simulink model "Silva22211767SL"  (R2025b)
settings: Solver=ode15s  StartTime=0.0  StopTime=100  RelTol=1e-3
settings Model: Creator=karla  LastModifiedBy=karla
settings DataIOCC: ReturnWorkspaceOutputs=off  TimeSaveName=t

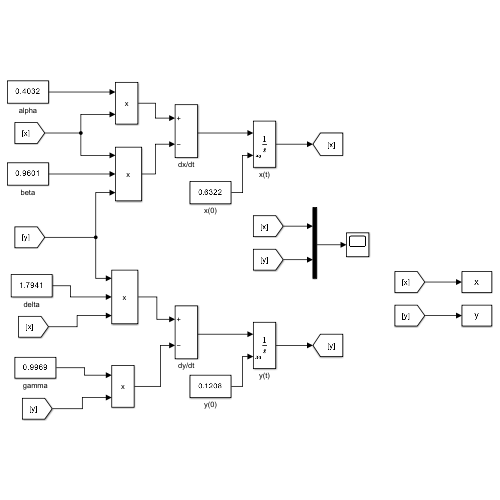
[thumbnail: Simulink's stored preview of the top-level diagram]
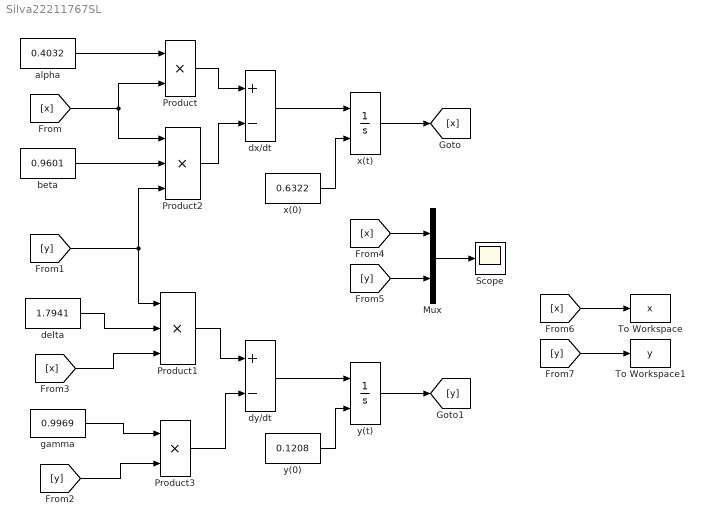
== system Silva22211767SL ==
  Mux : Mux  Inputs=2
  Product : Product
  Product1 : Product  Inputs=3
  Product2 : Product  Inputs=3
  Product3 : Product
  Scope : Scope
      settings: ActiveDisplayYMinimum=-0.19044498663156928  ActiveDisplayYMaximum=1.2600049250532
  To Workspace : ToWorkspace  VariableName=x  SampleTime=-1
  To Workspace1 : ToWorkspace  VariableName=y  SampleTime=-1
  alpha : Constant  Value=0.4032
  beta : Constant  Value=0.9601
  delta : Constant  Value=1.7941
  dx/dt : Sum  Inputs=+-
  dy/dt : Sum  Inputs=+-
  gamma : Constant  Value=0.9969
  x(0) : Constant  Value=0.6322
  x(t) : Integrator  InitialConditionSource=external
  y(0) : Constant  Value=0.1208
  y(t) : Integrator  InitialConditionSource=external
  wires:
  Product/1 -> dx/dt/1
  Product2/1 -> dx/dt/2
  Product1/1 -> dy/dt/1
  x(0)/1 -> x(t)/2
  y(0)/1 -> y(t)/2
  y(t)/1 -> [y]
  x(t)/1 -> [x]
  alpha/1 -> Product/1
  beta/1 -> Product2/2
  [x] -> Product2/1, Product/2
  [y] -> Product1/1, Product2/3
  Product3/1 -> dy/dt/2
  gamma/1 -> Product3/1
  delta/1 -> Product1/2
  [y] -> Product3/2
  [x] -> Product1/3
  dx/dt/1 -> x(t)/1
  dy/dt/1 -> y(t)/1
  Mux/1 -> Scope/1
  [x] -> Mux/1
  [y] -> Mux/2
  [y] -> To Workspace1/1
  [x] -> To Workspace/1
